simulink subsystem "Back_EMP"  (R2023a)
settings: Solver=VariableStepAuto  StartTime=0.0  StopTime=10.0  RelTol=1e-3
model mask{C_omega=C_omega}
  mask prompts: C_omega "Mechanical coef for velocity"
settings Model: Creator=ПК  LastModifiedBy=ПК

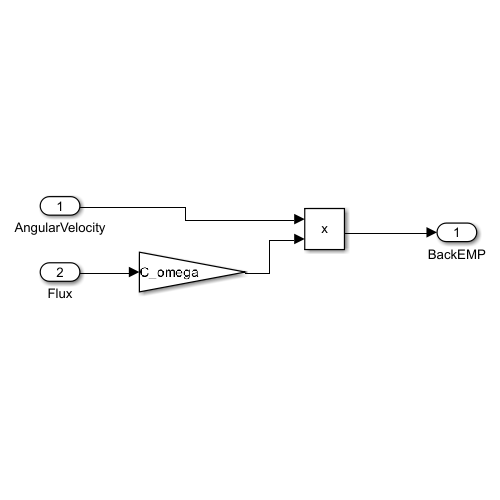
[thumbnail: Simulink's stored preview of the top-level diagram]
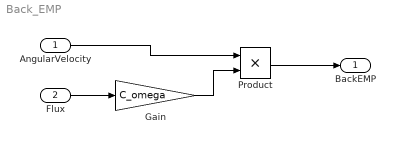
== system Back_EMP ==
  AngularVelocity : Inport
  Flux : Inport  Port=2
  Gain : Gain  Gain=C_omega
  Product : Product
  BackEMP : Outport
  wires:
  Flux/1 -> Gain/1
  Gain/1 -> Product/2
  AngularVelocity/1 -> Product/1
  Product/1 -> BackEMP/1
